simulink model "UAVFormation"  (R2021a)
settings: Solver=FixedStepAuto  StartTime=0.0  StopTime=150  FixedStep=0.1  RelTol=1e-3
(part 2 of 2)

== matlab function UAVFormation/MATLAB Function4 ==
  data: U1 input; w1 output; U2 input; U3 input; U4 input; w2 output; w3 output; w4 output
function [w1,w2,w3,w4] = fcn(U1,U2,U3,U4)
    CT = 1.116e-5; dCT = 0.225*CT;
    matrixA = [CT,CT,CT,CT;0,CT,0,-CT;-CT,0,CT,0;-dCT,dCT,-dCT,dCT];
    w_2 = inv(matrixA)*[U1,U2,U3,U4]';
    w1 = sqrt(abs(w_2(1))); w2 = sqrt(abs(w_2(2)));
    w3 = sqrt(abs(w_2(3))); w4 = sqrt(abs(w_2(4)));
end
